simulink model "chap6_3sim"  (Simulink 8.3)
settings: Solver=ode45  StartTime=0.0  StopTime=20  FixedStep=0.001  RelTol=1e-3
settings Model: Creator=hp  LastModifiedBy=Administrator  ExtModeTrigMode=oneshot  ExtModeArmWhenConnect=off
settings DataIOCC: LimitDataPoints=off  SignalLoggingName=sigsOut
settings OptimizationCC: BooleanDataType=off  ExpressionDepthLimit=2147483647  InitFltsAndDblsToZero=on
settings DebuggingCC: SaveWithParameterizedLinksMsg=none  SignalResolutionControl=TryResolveAllWithWarning  SolverPrmCheckMsg=none  MultiTaskDSMMsg=warning  MultiTaskCondExecSysMsg=none  FcnCallInpInsideContextMsg=UseLocalSettings
settings HardwareCC: TargetUnknown=on
settings RTWCC: IncludeERTFirstTime=on
settings GRTTargetCC: TargetFcnLib=ansi_tfl_tmw.mat

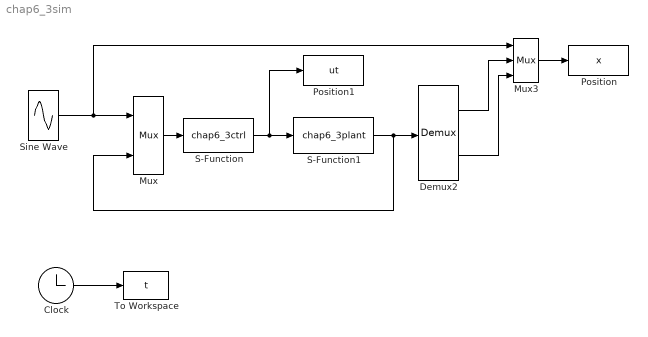
== system chap6_3sim ==
  Clock : Clock
  Demux2 : Demux  Outputs=2
  Mux : Mux  Inputs=2
  Mux3 : Mux  Inputs=3
  Position : ToWorkspace  VariableName=x  SampleTime=-1
  Position1 : ToWorkspace  VariableName=ut  SampleTime=-1
  S-Function : S-Function  FunctionName=chap6_3ctrl  EnableBusSupport=off
  S-Function1 : S-Function  FunctionName=chap6_3plant  EnableBusSupport=off
  Sine Wave : Sin  SampleTime=0
  To Workspace : ToWorkspace  VariableName=t  SampleTime=-1
  wires:
  Mux/1 -> S-Function/1
  Mux3/1 -> Position/1
  S-Function/1 -> Position1/1, S-Function1/1
  Demux2/1 -> Mux3/2
  S-Function1/1 -> Demux2/1, Mux/2
  Clock/1 -> To Workspace/1
  Sine Wave/1 -> Mux3/1, Mux/1
  Demux2/2 -> Mux3/3
